simulink model "VisionModel_v16"  (Simulink 7.6)
settings: Solver=FixedStepDiscrete  StartTime=0.0  StopTime=0  RelTol=1e-3
values from neighbouring files (symbols this model uses):
  Buoy_Max_Eccentricity = 1.2    [VisionConstants.m]
  Buoy_Max_Extent = 0.9    [VisionConstants.m]
  Buoy_Min_Eccentricity = 0    [VisionConstants.m]
  Buoy_Min_Extent = 0.1    [VisionConstants.m]
  Down_Camera_Dimensions = [120 160]    [VisionConstants.m]
  Forward_Camera_Dimensions = [160 120]    [VisionConstants.m]
undefined symbols (not defined in the file or in its folder): Forward_Fov, Rec, SDTV
libraries: vipconversions x8, vipgeotforms x6, viptextngfix x6, viptransforms x4, vipanalysis x3
(part 2 of 4)

== system VisionModel_v16/ColorSelect/torpedo ==
  Action Port : ActionPort  ActionType=elseif
  ColorFilter1 : Constant  Value=[0 0 1 1 0 0 0]  SampleTime=-1
  OutputSegmentedImage1 : Constant  SampleTime=-1
  ColorFilter : Outport  OutDataTypeStr=double
  OutputSegmentedImage : Outport  Port=2  OutDataTypeStr=double
  wires:
  OutputSegmentedImage1/1 -> OutputSegmentedImage/1
  ColorFilter1/1 -> ColorFilter/1

== system VisionModel_v16/ColorSelect/validation_gate ==
  Action Port : ActionPort  ActionType=then
  ColorFilter1 : Constant  Value=[0 1 0 0 1 0 0]  SampleTime=-1
  OutputSegmentedImage1 : Constant  SampleTime=-1
  ColorFilter : Outport  OutDataTypeStr=double
  OutputSegmentedImage : Outport  Port=2  OutDataTypeStr=double
  wires:
  ColorFilter1/1 -> ColorFilter/1
  OutputSegmentedImage1/1 -> OutputSegmentedImage/1

== system VisionModel_v16/L_detector/If Action Subsystem ==
  R_in : Inport
  G_in : Inport  Port=2
  B_in : Inport  Port=3
  which_camera : Inport  Port=4
  x_in : Inport  Port=5
  y_in : Inport  Port=6
  z_in : Inport  Port=7
  Camera_Dimensions : Inport  Port=8
  Action Port : ActionPort  ActionType=then
  Draw Target : viptextngfix/Draw Markers  DialogController=vipDDGCreate  DialogControllerArgs=DataTag8  shape=X-mark  size=7  fill=off  fillClrSource=Specify via dialog  display=User-specified value  intensity=200  color=[1 0 0]  opacity=0.6  viewport=Entire image  antialiasing=off  inType=Obsolete  imagePorts=Separate color signals  prodOutputMode=Binary point scaling  prodOutputWordLength=32  prodOutputFracLength=14  memoryMode=Specify word length  memoryWordLength=16  memoryFracLength=15  roundingMode=Floor  overflowMode=off
  Transform Coordinates3 : Stateflow chart  TreatAsAtomicUnit=on
  R_out : Outport  OutDataTypeStr=double
  G_out : Outport  Port=2  OutDataTypeStr=double
  B_out : Outport  Port=3  OutDataTypeStr=double
  wires:
  which_camera/1 -> Transform Coordinates3/1(which_camera)
  x_in/1 -> Transform Coordinates3/2(x_in)
  y_in/1 -> Transform Coordinates3/3(y_in)
  z_in/1 -> Transform Coordinates3/4(z_in)
  Camera_Dimensions/1 -> Transform Coordinates3/5(Camera_Dimensions)
  Draw Target/1 -> R_out/1
  Transform Coordinates3/1(points) -> Draw Target/4
  Draw Target/2 -> G_out/1
  Draw Target/3 -> B_out/1
  R_in/1 -> Draw Target/1
  G_in/1 -> Draw Target/2
  B_in/1 -> Draw Target/3

== system VisionModel_v16/buoy_detector/If Action Subsystem ==
  R_in : Inport
  G_in : Inport  Port=2
  B_in : Inport  Port=3
  which_camera : Inport  Port=4
  x_in : Inport  Port=5
  y_in : Inport  Port=6
  z_in : Inport  Port=7
  Camera_Dimensions : Inport  Port=8
  Action Port : ActionPort  ActionType=then
  Draw Target : viptextngfix/Draw Markers  DialogController=vipDDGCreate  DialogControllerArgs=DataTag9  shape=X-mark  size=7  fill=off  fillClrSource=Specify via dialog  display=User-specified value  intensity=200  color=[1 0 0]  opacity=0.6  viewport=Entire image  antialiasing=off  inType=Obsolete  imagePorts=Separate color signals  prodOutputMode=Binary point scaling  prodOutputWordLength=32  prodOutputFracLength=14  memoryMode=Specify word length  memoryWordLength=16  memoryFracLength=15  roundingMode=Floor  overflowMode=off
  Transform Coordinates3 : Stateflow chart  TreatAsAtomicUnit=on
  R_out : Outport  OutDataTypeStr=double
  G_out : Outport  Port=2  OutDataTypeStr=double
  B_out : Outport  Port=3  OutDataTypeStr=double
  wires:
  which_camera/1 -> Transform Coordinates3/1(which_camera)
  x_in/1 -> Transform Coordinates3/2(x_in)
  y_in/1 -> Transform Coordinates3/3(y_in)
  z_in/1 -> Transform Coordinates3/4(z_in)
  Camera_Dimensions/1 -> Transform Coordinates3/5(Camera_Dimensions)
  Draw Target/1 -> R_out/1
  Draw Target/2 -> G_out/1
  Draw Target/3 -> B_out/1
  R_in/1 -> Draw Target/1
  G_in/1 -> Draw Target/2
  B_in/1 -> Draw Target/3
  Transform Coordinates3/1(points) -> Draw Target/4

== system VisionModel_v16/path_detector/If Action Subsystem ==
  R_in : Inport
  G_in : Inport  Port=2
  B_in : Inport  Port=3
  which_camera : Inport  Port=4
  x_in : Inport  Port=5
  y_in : Inport  Port=6
  z_in : Inport  Port=7
  Camera_Dimensions : Inport  Port=8
  Action Port : ActionPort  ActionType=then
  Draw Target : viptextngfix/Draw Markers  DialogController=vipDDGCreate  DialogControllerArgs=DataTag12  shape=X-mark  size=7  fill=off  fillClrSource=Specify via dialog  display=User-specified value  intensity=200  color=[1 0 0]  opacity=0.6  viewport=Entire image  antialiasing=off  inType=Obsolete  imagePorts=Separate color signals  prodOutputMode=Binary point scaling  prodOutputWordLength=32  prodOutputFracLength=14  memoryMode=Specify word length  memoryWordLength=16  memoryFracLength=15  roundingMode=Floor  overflowMode=off
  Transform Coordinates3 : Stateflow chart  TreatAsAtomicUnit=on
  R_out : Outport  OutDataTypeStr=double
  G_out : Outport  Port=2  OutDataTypeStr=double
  B_out : Outport  Port=3  OutDataTypeStr=double
  wires:
  which_camera/1 -> Transform Coordinates3/1(which_camera)
  x_in/1 -> Transform Coordinates3/2(x_in)
  y_in/1 -> Transform Coordinates3/3(y_in)
  z_in/1 -> Transform Coordinates3/4(z_in)
  Camera_Dimensions/1 -> Transform Coordinates3/5(Camera_Dimensions)
  R_in/1 -> Draw Target/1
  G_in/1 -> Draw Target/2
  B_in/1 -> Draw Target/3
  Transform Coordinates3/1(points) -> Draw Target/4
  Draw Target/1 -> R_out/1
  Draw Target/2 -> G_out/1
  Draw Target/3 -> B_out/1

== system VisionModel_v16/torpedo/If Action Subsystem ==
  R_in : Inport
  G_in : Inport  Port=2
  B_in : Inport  Port=3
  which_camera : Inport  Port=4
  x_in : Inport  Port=5
  y_in : Inport  Port=6
  z_in : Inport  Port=7
  Camera_Dimensions : Inport  Port=8
  Action Port : ActionPort  ActionType=then
  Draw Target : viptextngfix/Draw Markers  DialogController=vipDDGCreate  DialogControllerArgs=DataTag13  shape=X-mark  size=7  fill=off  fillClrSource=Specify via dialog  display=User-specified value  intensity=200  color=[1 0 0]  opacity=0.6  viewport=Entire image  antialiasing=off  inType=Obsolete  imagePorts=Separate color signals  prodOutputMode=Binary point scaling  prodOutputWordLength=32  prodOutputFracLength=14  memoryMode=Specify word length  memoryWordLength=16  memoryFracLength=15  roundingMode=Floor  overflowMode=off
  Transform Coordinates3 : Stateflow chart  TreatAsAtomicUnit=on
  R_out : Outport  OutDataTypeStr=double
  G_out : Outport  Port=2  OutDataTypeStr=double
  B_out : Outport  Port=3  OutDataTypeStr=double
  wires:
  which_camera/1 -> Transform Coordinates3/1(which_camera)
  x_in/1 -> Transform Coordinates3/2(x_in)
  y_in/1 -> Transform Coordinates3/3(y_in)
  z_in/1 -> Transform Coordinates3/4(z_in)
  Camera_Dimensions/1 -> Transform Coordinates3/5(Camera_Dimensions)
  Draw Target/1 -> R_out/1
  Transform Coordinates3/1(points) -> Draw Target/4
  Draw Target/2 -> G_out/1
  Draw Target/3 -> B_out/1
  R_in/1 -> Draw Target/1
  G_in/1 -> Draw Target/2
  B_in/1 -> Draw Target/3

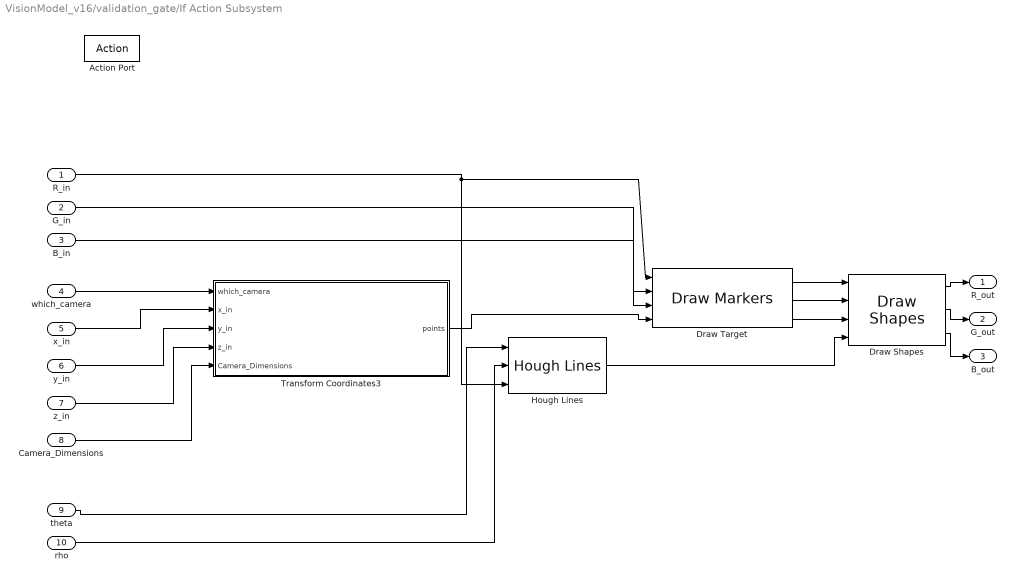
== system VisionModel_v16/validation_gate/If Action Subsystem ==
  R_in : Inport
  G_in : Inport  Port=2
  B_in : Inport  Port=3
  which_camera : Inport  Port=4
  x_in : Inport  Port=5
  y_in : Inport  Port=6
  z_in : Inport  Port=7
  Camera_Dimensions : Inport  Port=8
  theta : Inport  Port=9
  rho : Inport  Port=10
  Action Port : ActionPort  ActionType=then
  Draw Shapes : viptextngfix/Draw Shapes  DialogController=vipDDGCreate  DialogControllerArgs=DataTag16  shape=Lines  fill=off  fillClrSource=Specify via dialog  display=Black  intensity=200  color=[200 255 100]  opacity=0.6  viewport=Entire image  antialiasing=off  inType=Obsolete  imagePorts=Separate color signals  prodOutputMode=Binary point scaling  prodOutputWordLength=32  prodOutputFracLength=14  memoryMode=Specify word length  memoryWordLength=16  memoryFracLength=15  roundingMode=Floor  overflowMode=off
  Draw Target : viptextngfix/Draw Markers  DialogController=vipDDGCreate  DialogControllerArgs=DataTag17  shape=X-mark  size=7  fill=off  fillClrSource=Specify via dialog  display=User-specified value  intensity=200  color=[1 0 0]  opacity=0.6  viewport=Entire image  antialiasing=off  inType=Obsolete  imagePorts=Separate color signals  prodOutputMode=Binary point scaling  prodOutputWordLength=32  prodOutputFracLength=14  memoryMode=Specify word length  memoryWordLength=16  memoryFracLength=15  roundingMode=Floor  overflowMode=off
  Hough Lines : viptransforms/Hough Lines  DialogController=vipDDGCreate  DialogControllerArgs=DataTag18  sineCompMethod=Trigonometric function  thetaRes=pi/180  firstCoeffMode=Specify word length  firstCoeffWordLength=16  firstCoeffFracLength=15  prodOutputMode=Binary point scaling  prodOutputWordLength=32  prodOutputFracLength=16  roundingMode=Nearest  overflowMode=on
  Transform Coordinates3 : Stateflow chart  TreatAsAtomicUnit=on
  R_out : Outport  OutDataTypeStr=double
  G_out : Outport  Port=2  OutDataTypeStr=double
  B_out : Outport  Port=3  OutDataTypeStr=double
  wires:
  which_camera/1 -> Transform Coordinates3/1(which_camera)
  x_in/1 -> Transform Coordinates3/2(x_in)
  y_in/1 -> Transform Coordinates3/3(y_in)
  z_in/1 -> Transform Coordinates3/4(z_in)
  Camera_Dimensions/1 -> Transform Coordinates3/5(Camera_Dimensions)
  Hough Lines/1 -> Draw Shapes/4
  Draw Shapes/1 -> R_out/1
  Draw Shapes/2 -> G_out/1
  Draw Shapes/3 -> B_out/1
  R_in/1 -> Hough Lines/3, Draw Target/1
  theta/1 -> Hough Lines/1
  rho/1 -> Hough Lines/2
  Draw Target/1 -> Draw Shapes/1
  Draw Target/2 -> Draw Shapes/2
  Draw Target/3 -> Draw Shapes/3
  G_in/1 -> Draw Target/2
  B_in/1 -> Draw Target/3
  Transform Coordinates3/1(points) -> Draw Target/4

== system VisionModel_v16/Blob_Analysis/IterativeSegmentation/Low Pass Filter ==
  R : Inport
  G : Inport  Port=2
  B : Inport  Port=3
  Low Pass Filter : Stateflow chart  TreatAsAtomicUnit=on
  Low Pass Filter1 : Stateflow chart  TreatAsAtomicUnit=on
  Low Pass Filter2 : Stateflow chart  TreatAsAtomicUnit=on
  R' : Outport
  G' : Outport  Port=2
  B' : Outport  Port=3
  wires:
  Low Pass Filter/1(Iout) -> R'/1
  Low Pass Filter2/1(Iout) -> B'/1
  Low Pass Filter1/1(Iout) -> G'/1
  B/1 -> Low Pass Filter2/1(I)
  G/1 -> Low Pass Filter1/1(I)
  R/1 -> Low Pass Filter/1(I)

== system VisionModel_v16/Blob_Analysis/IterativeSegmentation/Segmentation ==
  L : Inport
  a : Inport  Port=2
  b : Inport  Port=3
  DesiredBuoyColor13 : Constant  Value=35  SampleTime=-1
  Iter_Segment_Thresh : Constant  Value=30  SampleTime=-1
  LabSegmentation : Stateflow chart  TreatAsAtomicUnit=on
  Reference Color Selection : Stateflow chart  TreatAsAtomicUnit=on
  Resize : Subsystem
  LabelMatrix : Outport
  num_colors : Outport  Port=2
  ref_colors : Outport  Port=3
  wires:
  LabSegmentation/1(LabelMatrix) -> LabelMatrix/1
  Reference Color Selection/2(num_colors) -> LabSegmentation/5(num_colors), num_colors/1
  Reference Color Selection/1(ref_colors) -> ref_colors/1, LabSegmentation/4(ref_colors)
  Resize/3(Out3) -> Reference Color Selection/3(b)
  Resize/2(Out2) -> Reference Color Selection/2(a)
  Resize/1(Out1) -> Reference Color Selection/1(L)
  b/1 -> LabSegmentation/3(b), Resize/3(In3)
  a/1 -> LabSegmentation/2(a), Resize/2(In2)
  L/1 -> LabSegmentation/1(L), Resize/1(In1)
  Iter_Segment_Thresh/1 -> Reference Color Selection/4(Dist_Thresh)

== system VisionModel_v16/Blob_Analysis1/IterativeSegmentation/Low Pass Filter ==
  R : Inport
  G : Inport  Port=2
  B : Inport  Port=3
  Low Pass Filter : Stateflow chart  TreatAsAtomicUnit=on
  Low Pass Filter1 : Stateflow chart  TreatAsAtomicUnit=on
  Low Pass Filter2 : Stateflow chart  TreatAsAtomicUnit=on
  R' : Outport
  G' : Outport  Port=2
  B' : Outport  Port=3
  wires:
  Low Pass Filter/1(Iout) -> R'/1
  Low Pass Filter2/1(Iout) -> B'/1
  Low Pass Filter1/1(Iout) -> G'/1
  B/1 -> Low Pass Filter2/1(I)
  G/1 -> Low Pass Filter1/1(I)
  R/1 -> Low Pass Filter/1(I)

== system VisionModel_v16/Blob_Analysis1/IterativeSegmentation/Segmentation ==
  L : Inport
  a : Inport  Port=2
  b : Inport  Port=3
  DesiredBuoyColor13 : Constant  Value=35  SampleTime=-1
  Iter_Segment_Thresh : Constant  Value=35  SampleTime=-1
  LabSegmentation : Stateflow chart  TreatAsAtomicUnit=on
  Reference Color Selection : Stateflow chart  TreatAsAtomicUnit=on
  Resize : Subsystem
  LabelMatrix : Outport
  num_colors : Outport  Port=2
  ref_colors : Outport  Port=3
  wires:
  LabSegmentation/1(LabelMatrix) -> LabelMatrix/1
  Reference Color Selection/2(num_colors) -> LabSegmentation/5(num_colors), num_colors/1
  Reference Color Selection/1(ref_colors) -> ref_colors/1, LabSegmentation/4(ref_colors)
  Resize/3(Out3) -> Reference Color Selection/3(b)
  Resize/2(Out2) -> Reference Color Selection/2(a)
  Resize/1(Out1) -> Reference Color Selection/1(L)
  b/1 -> LabSegmentation/3(b), Resize/3(In3)
  a/1 -> LabSegmentation/2(a), Resize/2(In2)
  L/1 -> LabSegmentation/1(L), Resize/1(In1)
  Iter_Segment_Thresh/1 -> Reference Color Selection/4(Dist_Thresh)

== system VisionModel_v16/Blob_Analysis/IterativeSegmentation/Segmentation/Resize ==
  In1 : Inport
  In2 : Inport  Port=2
  In3 : Inport  Port=3
  Resize : vipgeotforms/Resize  DialogController=vipDDGCreate  DialogControllerArgs=DataTag0  specify=Number of output rows and columns  rfactor=[]  outCols=25  outRows=25  outRowsCols=[60 80]  interp_method=Bilinear  antialias=on  useROI=off  roiFlag=off  prodOutputMode=Binary point scaling  prodOutputWordLength=32  prodOutputFracLength=10  roundingMode=Nearest  overflowMode=on
  Resize1 : vipgeotforms/Resize  DialogController=vipDDGCreate  DialogControllerArgs=DataTag1  specify=Number of output rows and columns  rfactor=[200 150]  outCols=25  outRows=25  outRowsCols=[60 80]  interp_method=Bilinear  antialias=on  useROI=off  roiFlag=off  prodOutputMode=Binary point scaling  prodOutputWordLength=32  prodOutputFracLength=10  roundingMode=Nearest  overflowMode=on
  Resize2 : vipgeotforms/Resize  DialogController=vipDDGCreate  DialogControllerArgs=DataTag2  specify=Number of output rows and columns  rfactor=[200 150]  outCols=25  outRows=25  outRowsCols=[60 80]  interp_method=Bilinear  antialias=on  useROI=off  roiFlag=off  prodOutputMode=Binary point scaling  prodOutputWordLength=32  prodOutputFracLength=10  roundingMode=Nearest  overflowMode=on
  Out1 : Outport
  Out2 : Outport  Port=2
  Out3 : Outport  Port=3
  wires:
  Resize2/1 -> Out3/1
  In3/1 -> Resize2/1
  Resize1/1 -> Out2/1
  In2/1 -> Resize1/1
  Resize/1 -> Out1/1
  In1/1 -> Resize/1

== system VisionModel_v16/Blob_Analysis1/IterativeSegmentation/Segmentation/Resize ==
  In1 : Inport
  In2 : Inport  Port=2
  In3 : Inport  Port=3
  Resize : vipgeotforms/Resize  DialogController=vipDDGCreate  DialogControllerArgs=DataTag3  specify=Number of output rows and columns  rfactor=[]  outCols=25  outRows=25  outRowsCols=[60 80]  interp_method=Bilinear  antialias=on  useROI=off  roiFlag=off  prodOutputMode=Binary point scaling  prodOutputWordLength=32  prodOutputFracLength=10  roundingMode=Nearest  overflowMode=on
  Resize1 : vipgeotforms/Resize  DialogController=vipDDGCreate  DialogControllerArgs=DataTag4  specify=Number of output rows and columns  rfactor=[200 150]  outCols=25  outRows=25  outRowsCols=[60 80]  interp_method=Bilinear  antialias=on  useROI=off  roiFlag=off  prodOutputMode=Binary point scaling  prodOutputWordLength=32  prodOutputFracLength=10  roundingMode=Nearest  overflowMode=on
  Resize2 : vipgeotforms/Resize  DialogController=vipDDGCreate  DialogControllerArgs=DataTag5  specify=Number of output rows and columns  rfactor=[200 150]  outCols=25  outRows=25  outRowsCols=[60 80]  interp_method=Bilinear  antialias=on  useROI=off  roiFlag=off  prodOutputMode=Binary point scaling  prodOutputWordLength=32  prodOutputFracLength=10  roundingMode=Nearest  overflowMode=on
  Out1 : Outport
  Out2 : Outport  Port=2
  Out3 : Outport  Port=3
  wires:
  Resize2/1 -> Out3/1
  In3/1 -> Resize2/1
  Resize1/1 -> Out2/1
  In2/1 -> Resize1/1
  Resize/1 -> Out1/1
  In1/1 -> Resize/1

== matlab function buoy_detector/If Action Subsystem/Transform Coordinates3 ==
  data: which_camera input double; x_in input double; y_in input double; z_in input double; Camera_Dimensions input double; points output double
function points = transform_G2L(which_camera, x_in, y_in, z_in, Camera_Dimensions)
% This function, "transform Global to Local coordinates," transforms
%   global coordinates that are sent to the controller into local
%   coordinates that can be displayed over images.
%
% 5-29-11
%
% Input
%   x_in, y_in, z_in = vectors of points in global (vehicle-centered)
%     coordinate system
%   bw_image_in = a 2-D array of pixel values (used only to extract image
%     size)
%   which_camera = selects which camera for relative coordinates
%                = 0 -> Forward camera
%                = 1 -> Down camera
%
% Output
%   r_out, c_out = row, column pairs in local coordinate system

rows = Camera_Dimensions(1);
cols = Camera_Dimensions(2);
if( which_camera == 0 )
    points = [z_in + floor(rows/2);
              y_in + floor(cols/2)];
else
    points = [floor(rows/2) - x_in;
              y_in + floor(cols/2)];
end


return

== matlab function torpedo/Decide which target to follow ==
  data: target_select output double; maintain_heading output double; target_y output double; centroids input double; id input double; which_color input double; target_z output double; target_yaw output double; target_detected output double; fire_authorization output double
function [target_select, maintain_heading, target_y, target_z, target_yaw, target_detected, fire_authorization]= determine_target(centroids, id, which_color)
% Decide which target to shoot at, based on which color is wanted.
%
% Input
%
% Output
%


% Initialize


%
target_select = 1;
maintain_heading = 0;
target_y = 0;
target_z = 0;
target_yaw = 0;
target_detected = 0;
fire_authorization = 0;

== matlab function torpedo/Analyze LabelMatrix for Targets ==
  data: centroids output double; blob_count input double; blob_hues input double; blob_centroids input double; blob_eccentricity input double; blob_extent input double; Min_Eccent input double; Max_Eccent input double; Min_Extent input double; Max_Extent input double; id output double
function [centroids, id]  = Target_Extraction(blob_count, blob_hues, blob_centroids, blob_eccentricity, blob_extent, Min_Eccent, Max_Eccent, Min_Extent, Max_Extent)
% This function takes in vectors representing blobs present in the image,
%   and returns information about how many and what kind of buoys are
%   present.
%
% Input
%   blob_count = integer number of blobs in image
%   blob_hues = Nx1 vector of hues of blobs in image
%   blob_centroids = Nx2 matrix of x-y pairs of blob centroid locations
%   blob_eccentricity = Nx1 vector of blob eccentricites
%   blob_extent = Nx1 vector of blob extents
%
%   Buoy_Count_Min = integer; minimum number of buoys searched for in an
%     image (mission/controls needs requires this option)
%   Buoy_Count_Max = maximum number of buoys allowed per image; arbitrary
%     limit
%   Min_Hue,Max_Hue = Nx1 limits on valid buoy hues; hue is between 0 and 1
%   Min_Eccent,Max_Eccent = scalar limits on buoy eccentricity
%   Min_Extent,Max_Extent = scalar limits on buoy extent
%
% Output
%   successive_valid_image_count = integer value of the number of times an
%     image with more than Min_Num_Buoys is processed; persistant between
%     function calls, so that the number of successive images containing
%     at least Min_Num_Buoys buoys is tracked
%   buoy_count = integer number of buoys in image
%   buoy_hues = Nx1 vector of buoy colors
%   buoy_centroids = Nx2 matrix of x-y pairs of buoy centroid locations

centroids = 0;
id = 0;


%{



% Initialize
%persistent successive_valid_image_count;
buoy_count = double(0);

%debug
%successive_valid_image_count = 0;
Buoy_Count_Max = 50;


%/debug
buoy_hues = double(zeros(Buoy_Count_Max,1));
buoy_centroids = double(-500.*ones(Buoy_Count_Max,2));  % Initialize to points clearly not located in image

buoy_id = double(-1.*ones(Buoy_Count_Max,1));
Buoy_Hue_HalfRange = 10;
Buoy1_Hue = 30;
Buoy2_Hue = 80;
Buoy3_Hue = 15;

% Loop through blobs, and analyze and extract buoy information
for i = 1:blob_count
    
    % Convert Lab to XYZ
%    R = buoy_hues(i);
%    G = buoy_hues(i);
%    B = buoy_hues(i);
    
    L = blob_hues(:,1); %refcolors(LabelMatrix(1,1,1));
    a = blob_hues(:,2);
    b = blob_hues(:,3);
    
    var_Y = L./10;
    var_X = ( a./17.5 ).*( L./10 );
    var_Z = ( b./7 ).*( L./10 );
    
    Y = var_Y.^2;
    X = ( var_X + Y )./1.02;
    Z = -( var_Z - Y )./0.847;
    
    % Convert XYZ to RGB
    var_X = X./100;        %X from 0 to  95.047      (Observer = 2 degrees, Illuminant = D65)
    var_Y = Y./100;        %Y from 0 to 100.000
    var_Z = Z./100;        %Z from 0 to 108.883
    
    var_R = var_X.*3.2406 + var_Y.*(-1.5372) + var_Z.* -0.4986;
    var_G = var_X .* -0.9689 + var_Y .*  1.8758 + var_Z.*  0.0415;
    var_B = var_X .*  0.0557 + var_Y .* -0.2040 + var_Z .*  1.0570;
    
    var_R = ( var_R > 0.0031308 ).*( 1.055.*( var_R.^( 1./2.4 ) ) - 0.055 ) + ( var_R <= 0.0031308 ).*(12.92.*var_R);
    var_G = ( var_G > 0.0031308 ).*( 1.055.*( var_G.^( 1./2.4 ) ) - 0.055 ) + ( var_G <= 0.0031308 ).*( var_G <= 12.92.*var_G );
    var_B = ( var_B > 0.0031308 ).*( 1.055 .* ( var_B .^ ( 1 ./ 2.4 ) ) - 0.055 ) + ( var_B <= 0.0031308 ).*( 12.92 .* var_B );
    
    R = var_R .* 255;
    G = var_G .* 255;
    B = var_B .* 255;
    
    % Convert RGB to HSV
    var_R = ( R ./ 255 );  % RGB from 0 to 255
    var_G = ( G ./ 255 );
    var_B = ( B ./ 255 );
    
    var_Min = min( [var_R, var_G, var_B], [], 2 );  % Min. value of RGB
    var_Max = max( [var_R, var_G, var_B], [], 2 );  % Max. value of RGB
    del_Max = var_Max - var_Min;  % Delta RGB value
    
    V = var_Max;
    
%    H = (del_Max != 0).*(  );
%    S = (del_Max != 0).*( del_Max./var_Max );
    if ( max(abs(del_Max == 0)) );  % This is a gray, no chroma...
        H = zeros(size(var_R));  % HSV results from 0 to 1
        S = zeros(size(var_R));
    else  % Chromatic data...
        
        S = del_Max ./ var_Max;
        
        del_R = ( ( ( var_Max - var_R ) ./ 6 ) + ( del_Max ./ 2 ) ) ./ del_Max;
        del_G = ( ( ( var_Max - var_G ) ./ 6 ) + ( del_Max ./ 2 ) ) ./ del_Max;
        del_B = ( ( ( var_Max - var_B ) ./ 6 ) + ( del_Max ./ 2 ) ) ./ del_Max;
        
        
        H = ( var_R == var_Max ).*( del_B - del_G ) + ( var_G == var_Max ).*( ( 1 ./ 3 ) + del_R - del_B ) + ( var_B == var_Max ).*( ( 2 ./ 3 ) + del_G - del_R );
        H = ( H < 0 ).*( H + 1 ) + ( H > 1 ).*( H - 1 );
        
        
%{        
        if( var_R == var_Max )
            H = del_B - del_G;
        elseif( var_G == var_Max )
            H = ( 1 ./ 3 ) + del_R - del_B;
        elseif( var_B == var_Max )
            H = ( 2 ./ 3 ) + del_G - del_R;
        else
            H = 0;
        end
        
        if( H < 0 )
            H = H + 1;
        end
        if( H > 1 )
            H = H - 1;
        end
%}        
    end
    
    
    
    
    
    
    
    
    
    % Store buoy information if blob conditions are met
    %   Conditions: 1) Blob eccentricity is within specified range
    %               2) Blob extent is within specified range
    %               3) Blob hue is within specified range for several buoy
    %                 types
    if( (blob_eccentricity(i)>=Min_Eccent) && (blob_eccentricity(i)<=Max_Eccent) && (blob_extent(i)>=Min_Extent) && (blob_extent(i)<=Max_Extent) )
        
        %if( (blob_hues(i)>=Buoy1_Hue-Buoy_Hue_HalfRange) && (blob_hues(i)<=Buoy1_Hue+Buoy_Hue_HalfRange) )
            buoy_count = buoy_count + 1;
            buoy_hues(buoy_count) = blob_hues(i);
            buoy_id(buoy_count) = 1;
            buoy_centroids(buoy_count,1) = blob_centroids(i,1);
            buoy_centroids(buoy_count,2) = blob_centroids(i,2);
        %end
        if( (blob_hues(i)>=Buoy2_Hue-Buoy_Hue_HalfRange) && (blob_hues(i)<=Buoy2_Hue+Buoy_Hue_HalfRange) )
            buoy_count = buoy_count + 1;
            buoy_hues(buoy_count) = blob_hues(i);
            buoy_id(buoy_count) = 2;
            buoy_centroids(buoy_count,1) = blob_centroids(i,1);
            buoy_centroids(buoy_count,2) = blob_centroids(i,2);
        end
        if( (blob_hues(i)>=Buoy3_Hue-Buoy_Hue_HalfRange) && (blob_hues(i)<=Buoy3_Hue+Buoy_Hue_HalfRange) )
            buoy_count = buoy_count + 1;
            buoy_hues(buoy_count) = blob_hues(i);
            buoy_id(buoy_count) = 3;
            buoy_centroids(buoy_count,1) = blob_centroids(i,1);
            buoy_centroids(buoy_count,2) = blob_centroids(i,2);
        end
    end
    
end


% Resize output arrays
%buoy_hues = buoy_hues(1:buoy_count);
%buoy_centroids = buoy_centroids(1:buoy_count,:);
%buoy_id = ;




%}



return

== matlab function buoy_detector/Shape_Analysis ==
  data: buoy_centroids output double; buoy_count output double; blob_hues input double; blob_centroids input double; blob_eccentricity input double; blob_extent input double; blob_count input double; blob_colors input double; Min_Eccent input double; Max_Eccent input double; Min_Extent input double; Max_Extent input double; buoy_colors output double
function [buoy_centroids, buoy_count, buoy_colors] = shape_analysis(blob_hues, blob_centroids, blob_eccentricity, blob_extent, blob_count, blob_colors, Min_Eccent, Max_Eccent, Min_Extent, Max_Extent)
% This function takes in vectors representing blobs present in the image,
%   and returns information about how many and what kind of buoys are
%   present. Buoys are identified by shape only.
%
% Input
%   blob_hues = Nx3 vector of hues of blobs in image (values are Lab
%     components)
%   blob_centroids = Nx2 matrix of x-y pairs of blob centroid locations
%   blob_eccentricity = Nx1 vector of blob eccentricites
%   blob_extent = Nx1 vector of blob extents
%   blob_count = integer number of blobs in image
%
%   Min_Hue,Max_Hue = Nx1 limits on valid buoy hues; hue is between 0 and 1
%   Min_Eccent,Max_Eccent = scalar limits on buoy eccentricity
%   Min_Extent,Max_Extent = scalar limits on buoy extent
%
%   Buoy_Count_Max = maximum number of buoys that will be analyzed
%
% Output
%   buoy_hues = Nx1 vector of buoy colors
%   buoy_centroids = Nx2 matrix of x-y pairs of buoy centroid locations
%   buoy_count = integer number of buoys found in image
%   buoy_colors = 1xN vector of buoy colors identified by blob analysis


% Initialize
Buoy_Count_Max = 50;
buoy_hues = double(zeros(Buoy_Count_Max,3));
buoy_centroids = double(-500.*ones(2,Buoy_Count_Max));  % Initialize to points clearly not located in image
buoy_count = double(0);
buoy_colors = zeros(1,Buoy_Count_Max);


% Loop through blobs, and extract information about blobs shaped like buoys
for i = 1:blob_count
    
    % Store buoy information if geometric conditions are met
    %   Conditions: 1) Blob eccentricity is within specified range
    %               2) Blob extent is within specified range
    if( (blob_eccentricity(i) >= Min_Eccent) && (blob_eccentricity(i) <= Max_Eccent) && (blob_extent(i) >= Min_Extent) && (blob_extent(i) <= Max_Extent) )
        
        buoy_count = buoy_count + 1;
        
        buoy_hues(buoy_count,1) = blob_hues(i,1);
        buoy_hues(buoy_count,2) = blob_hues(i,2);
        buoy_hues(buoy_count,3) = blob_hues(i,3);
        
        buoy_centroids(1,buoy_count) = blob_centroids(1,i);
        buoy_centroids(2,buoy_count) = blob_centroids(2,i);
%        buoy_centroids(buoy_count,1) = blob_centroids(i,1);
%        buoy_centroids(buoy_count,2) = blob_centroids(i,2);
        
        buoy_colors(buoy_count) = blob_colors(i);
        
    end
    
end


% If no buoy is identified, then loosen the shape restrictions and try again
if(buoy_count == 0)
    scale = 1.2;
    eccent_diff = scale*.5*(Max_Eccent - Min_Eccent);
    eccent_c = scale*.5*(Max_Eccent + Min_Eccent);
    extent_diff = .5*(Max_Extent - Min_Extent);
    extent_c = .5*(Max_Extent + Min_Extent);
    Min_Eccent = eccent_c - eccent_diff;
    Max_Eccent = eccent_c + eccent_diff;
    Min_Extent = extent_c - extent_diff;
    Max_Extent = extent_c + extent_diff;
    for i = 1:blob_count
        
        % Store buoy information if geometric conditions are met
        %   Conditions: 1) Blob eccentricity is within specified range
        %               2) Blob extent is within specified range
        if( (blob_eccentricity(i) >= Min_Eccent) && (blob_eccentricity(i) <= Max_Eccent) && (blob_extent(i) >= Min_Extent) && (blob_extent(i) <= Max_Extent) )
            
            buoy_count = buoy_count + 1;

            buoy_hues(buoy_count,1) = blob_hues(i,1);
            buoy_hues(buoy_count,2) = blob_hues(i,2);
            buoy_hues(buoy_count,3) = blob_hues(i,3);


            buoy_centroids(1,buoy_count) = blob_centroids(1,i);
            buoy_centroids(2,buoy_count) = blob_centroids(2,i);
            %buoy_centroids(buoy_count,1) = blob_centroids(i,1);
            %buoy_centroids(buoy_count,2) = blob_centroids(i,2);
            
            buoy_colors(buoy_count) = blob_colors(i);
            
        end

    end
end



return

== matlab function torpedo/If Action Subsystem/Transform Coordinates3 ==
  data: which_camera input double; x_in input double; y_in input double; z_in input double; Camera_Dimensions input double; points output double
function points = transform_G2L(which_camera, x_in, y_in, z_in, Camera_Dimensions)
% This function, "transform Global to Local coordinates," transforms
%   global coordinates that are sent to the controller into local
%   coordinates that can be displayed over images.
%
% 5-29-11
%
% Input
%   x_in, y_in, z_in = vectors of points in global (vehicle-centered)
%     coordinate system
%   bw_image_in = a 2-D array of pixel values (used only to extract image
%     size)
%   which_camera = selects which camera for relative coordinates
%                = 0 -> Forward camera
%                = 1 -> Down camera
%
% Output
%   r_out, c_out = row, column pairs in local coordinate system

rows = Camera_Dimensions(1);
cols = Camera_Dimensions(2);
if( which_camera == 0 )
    points = [z_in + floor(rows/2);
              y_in + floor(cols/2)];
else
    points = [floor(rows/2) - x_in;
              y_in + floor(cols/2)];
end


return

== matlab function buoy_detector/Choose_Buoy ==
  data: buoy_centroids input double; buoy_count input double; buoy_colors input double; target_select output double; maintain_heading output double; targetY output double; targetZ output double; targetYaw output double; target_detected output double; which_color input double; Forward_Camera_Dimensions input double; Forward_Fov input double
function [target_select, maintain_heading, targetY, targetZ, targetYaw, target_detected] = choose_buoy(buoy_centroids, buoy_count, buoy_colors, which_color, Forward_Camera_Dimensions, Forward_Fov)
% This function takes in vectors representing buoys present in the image,
%   and decides which buoy to target.
%
% Input
%   buoy_hues = Nx3 matrix of Lab components for each buoy
%   buoy_centroids = 2xN matrix of x-y pairs of buoy centroids
%   buoy_count = number of buoys identified in the image
%   buoy_colors = 1xN vector of buoy color indices
%   a_range, b_range = 2xN matrix of lower/upper bounds on a, b for each
%     color
%   which_color = which buoy color should be targeted; integer value
%     represents:
%               1 -> White
%               2 -> Black
%               3 -> Blue
%               4 -> Red
%               5 -> Orange
%               6 -> Yellow
%               7 -> Green
%
% Output
%   target_select = input to MotionController.mdl, which selects which
%     camera to use
%   maintain_heading = instructs MotionController to strafe xor turn:
%                    = 0 -> Turn toward target (use targetYaw)
%                    = 1 -> Strafe to target (use targetY)
%   targetY, targetZ = position of buoy in absolute coordinates
%   targetYaw = relative, lateral angular displacement of buoy from
%     straight ahead (in degrees)
%   target_detected = informs the script that a buoy is being tracked


% Initialize
target_select = 1;
maintain_heading = 0;
targetY = 0;
targetZ = 0;
targetYaw = 0;
target_detected = 0;
rows = Forward_Camera_Dimensions(1);
cols = Forward_Camera_Dimensions(2);

%{
% Classify each buoy by color
for i = 1:buoy_count
    
    a = buoy_hues(i, 2);
    b = buoy_hues(i, 3);
    
    % Note that colors 1 and 2 are black and white, resp. and do not have
    %   useful ranges in the a and b color components
    for col = 3:max_num_colors
        if( a >= a_range(1,col) && a <= a_range(2,col) && b >= b_range(1,col) && b <= b_range(2,col) )
            buoy_colors(i) = col;
            break;
        end
    end
    
end
%}




% Examine buoys from left to right; if one has the correct color, then
%   target it; else do not recognize a target
for i = 1:buoy_count
    if( buoy_colors(i) == which_color )
        targetY = buoy_centroids(2,i) - floor(cols/2);
        targetZ = buoy_centroids(1,i) - floor(rows/2);
        targetYaw = Forward_Fov*(targetY/cols);
        target_detected = 1;
        break;
    else
    end
end


% If no buoy was targeted, then pick one of the remaining buoys to target
if(target_detected == 0)
    targetY = buoy_centroids(2,1) - floor(cols/2);
    targetZ = buoy_centroids(1,1) - floor(rows/2);
    targetYaw = Forward_Fov*(targetY/cols);
end







%{


buoy_hues = double(zeros(Buoy_Count_Max,1));
buoy_centroids = double(-500.*ones(Buoy_Count_Max,2));  % Initialize to points clearly not located in image

buoy_id = double(-1.*ones(Buoy_Count_Max,1));
Buoy_Hue_HalfRange = 10;
Buoy1_Hue = 30;
Buoy2_Hue = 80;
Buoy3_Hue = 15;

% Loop through blobs, and analyze and extract buoy information
for i = 1:blob_count
    
    % Convert Lab to XYZ
%    R = buoy_hues(i);
%    G = buoy_hues(i);
%    B = buoy_hues(i);
    
    L = blob_hues(:,1); %refcolors(LabelMatrix(1,1,1));
    a = blob_hues(:,2);
    b = blob_hues(:,3);
    
    var_Y = L./10;
    var_X = ( a./17.5 ).*( L./10 );
    var_Z = ( b./7 ).*( L./10 );
    
    Y = var_Y.^2;
    X = ( var_X + Y )./1.02;
    Z = -( var_Z - Y )./0.847;
    
    % Convert XYZ to RGB
    var_X = X./100;        %X from 0 to  95.047      (Observer = 2 degrees, Illuminant = D65)
    var_Y = Y./100;        %Y from 0 to 100.000
    var_Z = Z./100;        %Z from 0 to 108.883
    
    var_R = var_X.*3.2406 + var_Y.*(-1.5372) + var_Z.* -0.4986;
    var_G = var_X .* -0.9689 + var_Y .*  1.8758 + var_Z.*  0.0415;
    var_B = var_X .*  0.0557 + var_Y .* -0.2040 + var_Z .*  1.0570;
    
    var_R = ( var_R > 0.0031308 ).*( 1.055.*( var_R.^( 1./2.4 ) ) - 0.055 ) + ( var_R <= 0.0031308 ).*(12.92.*var_R);
    var_G = ( var_G > 0.0031308 ).*( 1.055.*( var_G.^( 1./2.4 ) ) - 0.055 ) + ( var_G <= 0.0031308 ).*( var_G <= 12.92.*var_G );
    var_B = ( var_B > 0.0031308 ).*( 1.055 .* ( var_B .^ ( 1 ./ 2.4 ) ) - 0.055 ) + ( var_B <= 0.0031308 ).*( 12.92 .* var_B );
    
    R = var_R .* 255;
    G = var_G .* 255;
    B = var_B .* 255;
    
    % Convert RGB to HSV
    var_R = ( R ./ 255 );  % RGB from 0 to 255
    var_G = ( G ./ 255 );
    var_B = ( B ./ 255 );
    
    var_Min = min( [var_R, var_G, var_B], [], 2 );  % Min. value of RGB
    var_Max = max( [var_R, var_G, var_B], [], 2 );  % Max. value of RGB
    del_Max = var_Max - var_Min;  % Delta RGB value
    
    V = var_Max;
    
%    H = (del_Max != 0).*(  );
%    S = (del_Max != 0).*( del_Max./var_Max );
    if ( max(abs(del_Max == 0)) );  % This is a gray, no chroma...
        H = zeros(size(var_R));  % HSV results from 0 to 1
        S = zeros(size(var_R));
    else  % Chromatic data...
        
        S = del_Max ./ var_Max;
        
        del_R = ( ( ( var_Max - var_R ) ./ 6 ) + ( del_Max ./ 2 ) ) ./ del_Max;
        del_G = ( ( ( var_Max - var_G ) ./ 6 ) + ( del_Max ./ 2 ) ) ./ del_Max;
        del_B = ( ( ( var_Max - var_B ) ./ 6 ) + ( del_Max ./ 2 ) ) ./ del_Max;
        
        
        H = ( var_R == var_Max ).*( del_B - del_G ) + ( var_G == var_Max ).*( ( 1 ./ 3 ) + del_R - del_B ) + ( var_B == var_Max ).*( ( 2 ./ 3 ) + del_G - del_R );
        H = ( H < 0 ).*( H + 1 ) + ( H > 1 ).*( H - 1 );
        
        
%{        
        if( var_R == var_Max )
            H = del_B - del_G;
        elseif( var_G == var_Max )
            H = ( 1 ./ 3 ) + del_R - del_B;
        elseif( var_B == var_Max )
            H = ( 2 ./ 3 ) + del_G - del_R;
        else
            H = 0;
        end
        
        if( H < 0 )
            H = H + 1;
        end
        if( H > 1 )
            H = H - 1;
        end
%}        
    end
    
    
    
    
    
    
    
    
    
    % Store buoy information if blob conditions are met
    %   Conditions: 1) Blob eccentricity is within specified range
    %               2) Blob extent is within specified range
    %               3) Blob hue is within specified range for several buoy
    %                 types
    if( (blob_eccentricity(i)>=Min_Eccent) && (blob_eccentricity(i)<=Max_Eccent) && (blob_extent(i)>=Min_Extent) && (blob_extent(i)<=Max_Extent) )
        
        %if( (blob_hues(i)>=Buoy1_Hue-Buoy_Hue_HalfRange) && (blob_hues(i)<=Buoy1_Hue+Buoy_Hue_HalfRange) )
            buoy_count = buoy_count + 1;
            buoy_hues(buoy_count) = blob_hues(i);
            buoy_id(buoy_count) = 1;
            buoy_centroids(buoy_count,1) = blob_centroids(i,1);
            buoy_centroids(buoy_count,2) = blob_centroids(i,2);
        %end
        if( (blob_hues(i)>=Buoy2_Hue-Buoy_Hue_HalfRange) && (blob_hues(i)<=Buoy2_Hue+Buoy_Hue_HalfRange) )
            buoy_count = buoy_count + 1;
            buoy_hues(buoy_count) = blob_hues(i);
            buoy_id(buoy_count) = 2;
            buoy_centroids(buoy_count,1) = blob_centroids(i,1);
            buoy_centroids(buoy_count,2) = blob_centroids(i,2);
        end
        if( (blob_hues(i)>=Buoy3_Hue-Buoy_Hue_HalfRange) && (blob_hues(i)<=Buoy3_Hue+Buoy_Hue_HalfRange) )
            buoy_count = buoy_count + 1;
            buoy_hues(buoy_count) = blob_hues(i);
            buoy_id(buoy_count) = 3;
            buoy_centroids(buoy_count,1) = blob_centroids(i,1);
            buoy_centroids(buoy_count,2) = blob_centroids(i,2);
        end
    end
    
end

% Resize output arrays
%buoy_hues = buoy_hues(1:buoy_count);
%buoy_centroids = buoy_centroids(1:buoy_count,:);
%buoy_id = ;

%}








return

== matlab function L_detector/Identify L-Obstacle ==
  data: target_select output double; maintain_heading output double; hough_table input double; target_y output double; target_z output double; target_yaw output double; target_detected output double; theta_in input double; rho_in input double; blob_area input double; blob_centroid input double; blob_major_axis input double; blob_orientation input double; blob_count input double; target_ratio_v input double; target_ratio_h input double; Forward_Camera_Dimensions input double; Forward_Fov input double
function [target_select, maintain_heading, target_y, target_z, target_yaw, target_detected] = validation_gate(hough_table, theta_in, rho_in, blob_area, blob_centroid, blob_major_axis, blob_orientation, blob_count, target_ratio_v, target_ratio_h, Forward_Camera_Dimensions, Forward_Fov)
%#eml
%{

1. Iteratively segment image
2. Obtain information about all blobs in image
3. Generate a bw image by filtering colors (thresholding)

3.5. Identify one appropriate horizontal and one appropriate vertical blob

4. Perform edge detection then Hough transform to bw image
5. Identify the most popular lines (any orientation) that are:
     a) Nearly colinear with blobs, and
     b) At approximately 90 degrees from each other

6. Target appropriately

%}




% This function attempts to identfiy the L-shaped obstacle, and returns
%   targeting information, and a true/false target_detected parameter.


% Initialize
target_select = 1;
target_found = 1;
maintain_heading = 0;
target_y = 0;
target_z = 0;
target_yaw = 0;
target_detected = 0;


% Only the (max_num_lines) with the most votes will be considered as
%   candidates for the gate
max_num_lines = 200;
[rho_length, theta_length] = size(hough_table);
rows = Forward_Camera_Dimensions(1);
cols = Forward_Camera_Dimensions(2);

image_area = rows*cols;
area_thresh = 0.8;  % Ratio of blob area to image area considered to imply the blob is actually background noise

% eps_rho must be at least as big as the gate leg diameter (units of
%   pixels)
eps_rho = .1*max(rows,cols);
% eps_theta is used to distinguish lines as "horizontal" or "vertical";
%   units are radians
eps_theta = 10*pi/180;

% These vectors contain the final two lines that compose the L-obstacle
rho_gate = zeros(1,2);
theta_gate = zeros(1,2);

% These vectors contain intermediate line information; as lines are
%   eliminated from these vectors, their values are set to zero
% Note that rho_in and theta_in are referred to by hough_table; they do not
%   constitute (rho,theta) pairs without hough_table. rho and theta,
%   however, do constitute (rho,theta) pairs.
rho = zeros(1,max_num_lines);
theta = zeros(1,max_num_lines);


% Identify the most popular max_num_lines lines
i_index = ones(1,max_num_lines);
j_index = ones(1,max_num_lines);

for m = 1:max_num_lines
    
    max_votes = 0;
    for i = 1:rho_length
        for j = 1:theta_length
            if( hough_table(i,j) > max_votes )
                i_index(m) = i;
                j_index(m) = j;
                max_votes = hough_table(i,j);
            end
        end
    end
    
    rho(m) = rho_in(i_index(m));
    theta(m) = theta_in(j_index(m));
    hough_table(i_index(m),j_index(m)) = 0;
    
end


% Correct orientations to vehicle coordinates
for j = 1:blob_count
    % theta_hold:
    %   -is between [-pi/2, +pi/2]
    % blob_orientation:
    %   -is potentially outside this range
    %   -needs to be corrected by pi/2 to get relative heading
    blob_orientation(j) = mod(pi - blob_orientation(j), pi) - pi/2;
end


% Determine the most popular lines which are nearly colinear to blobs
theta_hold = theta;
i_gate = zeros(2,2);  % Indices for line and blob, respectively
for g = 1:2
    
    found = 0;
    for i = 1:max_num_lines
        for j = 1:blob_count
            
            % Search for a match between one blob and one line
            condition1 = abs(theta_hold(i) - blob_orientation(j)) <= eps_theta;
            condition2 = blob_area(j)/image_area <= area_thresh;
            condition3 = theta_hold(i) ~= 1000 && blob_orientation(j) ~= 1000;
            c1 = blob_centroid(2,j);
            r1 = blob_centroid(1,j);
            c2 = rho(i)*cos(theta(i)) - r1 + c1*sin(theta(i));
            r2 = -cot(theta(i))*c2 + rho(i)/sin(theta(i));
            d = sqrt( (c2 - c1)^2 + (r2 - r1)^2 );
            condition4 = d <= eps_rho;
            if(condition1 && condition2 && condition3 && condition4)
                
                if(g == 1)
                    
                    % Determine the first gate element
                    i_gate(1,g) = i;
                    i_gate(2,g) = j;
                    
                else
                    
                    % Assume the first gate element was found correctly;
                    %   check that all other gate elements are at right
                    %   angles to the first
                    if( abs((pi/2) - abs(theta_hold(i) - theta_hold( i_gate(1,1) ))) <= eps_theta)
                        i_gate(1,g) = i;
                        i_gate(2,g) = j;
                    end
                    
                end
                
                theta_hold(i) = 1000;  % Invalid angle; do not want this line to be selected again
                blob_orientation(j) = 1000;
                found = 1;
                break;
            end
            
        end
        
        if(found == 1)
            break;
        end
    end
    
end


if( ~(i_gate(1) == 0 && i_gate(2) == 0) )
    
    % Sort elements of i_gate to place the vertical element in the first
    %   position, horizontal element in second position
    ihold = i_gate(1,1);
    jhold = i_gate(2,1);
    if( abs(theta( i_gate(1,1) )) > abs(theta( i_gate(1,2) )) )
        i_gate(1,1) = i_gate(1,2);
        i_gate(2,1) = i_gate(2,2);

        i_gate(1,2) = ihold;
        i_gate(2,2) = jhold;
    end


    % Assign appropriate gate information
    for g = 1:2
        rho_gate(g) = rho( i_gate(1,g) );
        theta_gate(g) = theta( i_gate(1,g) );
    end


    % Compute targeting information
    % Determine side lengths and distances for target
    length1 = blob_major_axis(i_gate(2,1));
    length2 = blob_major_axis(i_gate(2,2));
    d1 = target_ratio_v*length1;
    d2 = target_ratio_h*length2;

    phi1 = blob_orientation(i_gate(2,1));
    phi2 = blob_orientation(i_gate(2,2));
    theta1 = (pi/2) - phi1;
    theta2 = (pi/2) - phi2;

    r1 = blob_centroid(1,i_gate(2,1));
    c1 = blob_centroid(2,i_gate(2,1));
    r2 = blob_centroid(1,i_gate(2,2));
    c2 = blob_centroid(2,i_gate(2,2));

    rho1 = c1*sin(theta1) + r1*cos(theta1);
    rho2 = c2*sin(theta2) + r2*cos(theta2);

    r3 = (1/( cos(theta1)*sin(theta2) - cos(theta2)*sin(theta1) ))*( rho1*sin(theta2) - rho2*sin(theta1) );
    c3 = -cot(theta1)*r3 + rho1/sin(theta1);
    %r3 = (1/( sin(phi1)*cos(phi2) - sin(phi2)*cos(phi1) ))*( c2 - c1 + sin(pih1)*cos(phi2)*r1 - sin(phi2)*cos(phi1)*r2 );
    %c3 = r3*tan(phi1) + c1 - r1*tan(phi1);

    r4 = r3 - d1*cos(phi1);
    c4 = c3 + d1*sin(phi1);

    r5 = r3 + d2*sin(phi2);
    c5 = c3 + d2*cos(phi2);

    theta4 = theta1;
    theta5 = theta2;

    rho4 = c4*sin(theta4) + r4*cos(theta4);
    rho5 = c5*sin(theta5) + r5*cos(theta5);

    r6 = (1/( cos(theta4)*sin(theta5) - cos(theta5)*sin(theta4) ))*( rho4*sin(theta5) - rho5*sin(theta4) );
    c6 = -cot(theta4)*r6 + rho4/sin(theta4);
    
    target_detected = 1;
    
    % Transform target r, c to global coordinate system
    target_z = r6 - floor(rows/2);
    target_y = c6 - floor(cols/2);
    
    target_yaw = Forward_Fov*( target_y/cols );
    target_detected = 0;
    
else
    
    target_y = 0;
    target_z = 0;
    target_yaw = 0;
    target_detected = 0;
    
end


return
